simulink model "simple_model"  (R2024b)
settings: Solver=FixedStepAuto  StartTime=0.0  StopTime=10.0  FixedStep=T  RelTol=1e-3
settings Model: DataDictionary=wrapper2.sldd  Creator=maciej  LastModifiedBy=maciej

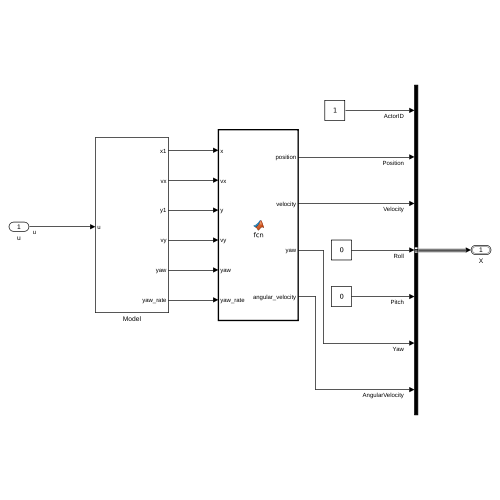
[thumbnail: Simulink's stored preview of the top-level diagram]
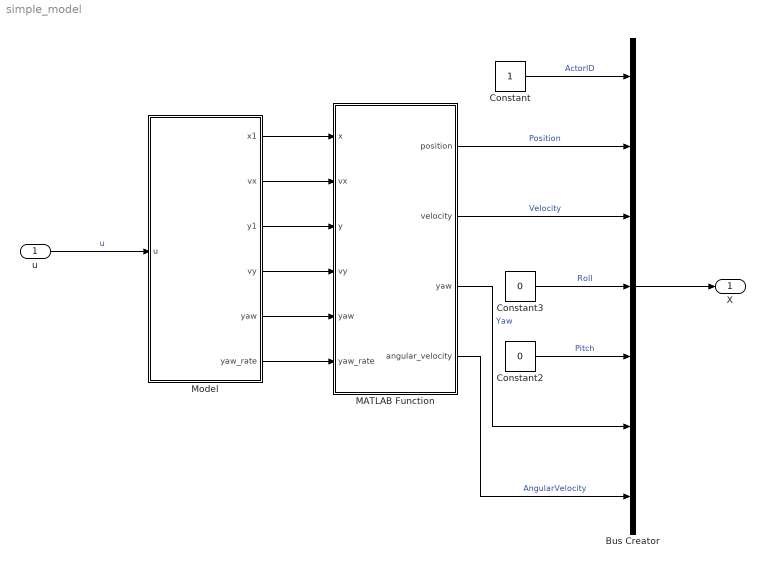
== system simple_model ==
  u : Inport
  Bus Creator : BusCreator  Inputs=7  OutDataTypeStr=Bus: EgoVehicle
  Constant : Constant
  Constant2 : Constant  Value=0
  Constant3 : Constant  Value=0
  MATLAB Function : MATLAB Function  TreatAsAtomicUnit=on
  Model : Subsystem
  X : Outport  OutDataTypeStr=Bus: EgoVehicle  PortDimensions=1
  wires:
  u/1 -> Model/1(u)  "u"
  Constant3/1 -> Bus Creator/4  "Roll"
  MATLAB Function/1(position) -> Bus Creator/2  "Position"
  MATLAB Function/2(velocity) -> Bus Creator/3  "Velocity"
  Bus Creator/1 -> X/1
  Constant2/1 -> Bus Creator/5  "Pitch"
  Constant/1 -> Bus Creator/1  "ActorID"
  MATLAB Function/4(angular_velocity) -> Bus Creator/7  "AngularVelocity"
  MATLAB Function/3(yaw) -> Bus Creator/6  "Yaw"
  Model/1(x1) -> MATLAB Function/1(x)
  Model/2(vx) -> MATLAB Function/2(vx)
  Model/3(y1) -> MATLAB Function/3(y)
  Model/4(vy) -> MATLAB Function/4(vy)
  Model/5(yaw) -> MATLAB Function/5("yaw ")
  Model/6(yaw_rate) -> MATLAB Function/6(yaw_rate)

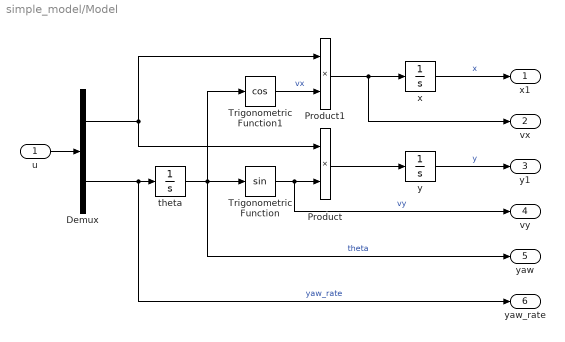
== system simple_model/Model ==
  u : Inport
  Demux : Demux  Outputs=2
  Product : Product
  Product1 : Product
  Trigonometric Function : Trigonometry
  Trigonometric Function1 : Trigonometry  Operator=cos
  theta : Integrator
  x : Integrator
  y : Integrator
  x1 : Outport
  vx : Outport  Port=2
  y1 : Outport  Port=3
  vy : Outport  Port=4
  yaw : Outport  Port=5
  yaw_rate : Outport  Port=6
  wires:
  theta/1 -> yaw/1, Trigonometric Function1/1, Trigonometric Function/1  "theta"
  y/1 -> y1/1  "y"
  Trigonometric Function/1 -> Product/2, vy/1  "vy"
  x/1 -> x1/1  "x"
  u/1 -> Demux/1
  Demux/2 -> yaw_rate/1, theta/1  "yaw_rate"
  Demux/1 -> Product/1, Product1/1
  Trigonometric Function1/1 -> Product1/2  "vx"
  Product1/1 -> vx/1, x/1
  Product/1 -> y/1

== matlab function simple_model/MATLAB Function ==
  data: x input; position output; velocity output; yaw output; angular_velocity output; vx input; y input; vy input; yaw input; yaw_rate input
function [position, velocity, yaw, angular_velocity] = fcn(x, vx, y, vy, yaw, yaw_rate)
    position = [x, y, 0];
    velocity = [vx, vy, 0];

    angular_velocity = [0, 0, yaw_rate];
end
